simulink model "IEEE34bus_v2019b_Phasor_DPL_ZIPload"  (R2019b)
settings: Solver=VariableStepAuto  StartTime=0.0  StopTime=100  FixedStep=Ts  RelTol=1e-3
InitFcn:
  | a=1; % Loading Factor
  | Ts=0.1;% For Delay Blocks in Voltage Regulator Controls
  | 
  | % Simulation data for the IEEE 34 Node Test Feeder model
  | mi2km = 1.60934;%  miles to km conversion
  | ft2km = 0.0003048; % feet to km conversion
  | ms2F = 1*1e-6/(2*pi*60);% microsiemens to Farads conversion
  | 
  | %% Configuration 300 - series reactance - ohm/mile
  | R_300 = [1.3368 0.2101 0.2130;0.2101 1.3238 0.2066;0.2130 0.2066 1.3294];
  | X_300 = [1.3343 0.5779 0.5015;0.5779 1.3569 0.4591;0.5015 0.4591 1.3471];
  | % charging susceptance - microsiemens/mile
  | B_300 = [5.3350 -1.5313 -0.9943;-1.5313 5.0979 -0.6212;-0.9943 -0.6212 4.8880];
  | 
  | R_300 = R_300/mi2km;
  | L_300 = (X_300/(2*pi*60))/mi2km;
  | C_300 =(B_300*ms2F)/mi2km;
  | 
  | %% Configuration 301 - series reactance - ohm/mile
  | R_301 = [1.9300 0.2327 0.2359;0.2327 1.9157 0.2288;0.2359 0.2288 1.9219];
  | X_301 = [1.4115 0.6442 0.5691;0.6442 1.4281 0.5238;0.5691 0.5238 1.4209];
  | % charging susceptance - microsiemens/mile
  | B_301 = [5.1207 -1.4364 -0.9402;-1.4364 4.9055 -0.5951;-0.9402 -0.5951 4.7154];
  | 
  | R_301 = R_301/mi2km;
  | L_301 = (X_301/(2*pi*60))/mi2km;
  | C_301 =(B_301*ms2F)/mi2km;
  | 
  | 
  | %% Configuration 302 - series reactance - ohm/mile
  | R_302 = [2.7995 0 0;0 0 0;0 0 0];
  | X_302 = [1.4855 0 0;0 0 0;0 0 0];
  | % charging susceptance - microsiemens/mile
  | B_302 = [4.2251 0 0;0 0 0;0 0 0];
  | 
  | R_302 = R_302/mi2km;
  | L_302 = (X_302/(2*pi*60))/mi2km;
  | C_302 =(B_302*ms2F)/mi2km;
  | 
  | %% Configuration 303 - series reactance - ohm/mile
  | R_303 = [0 0 0;0 2.7995 0;0 0 0];
  | X_303 = [0 0 0;0 1.4855 0;0 0 0];
  | % charging susceptance - microsiemens/mile
  | B_303 = [0 0 0;0 4.2251 0;0 0 0];
  | 
  | R_303 = R_303/mi2km;
  | L_303 = (X_303/(2*pi*60))/mi2km;
  | C_303 =(B_303*ms2F)/mi2km;
  | 
  | %% Configuration 303 - series reactance - ohm/mile
  | R_304 = [0 0 0;0 1.9217 0;0 0 0];
  | X_304 = [0 0 0;0 1.4212 0;0 0 0];
  | % charging susceptance - microsiemens/mile
  | B_304 = [0 0 0;0 4.3637 0;0 0 0];
  | 
  | R_304 = R_304/mi2km;
  | L_304 = (X_304/(2*pi*60))/mi2km;
  | C_304 =(B_304*ms2F)/mi2km;
undefined symbols (not defined in the file): find_system, j
libraries: powerlib x471, powerlib_meascontrol x22
(part 7 of 9)

== system IEEE34bus_v2019b_Phasor_DPL_ZIPload/Regulator 1/Single Phase SVR_B/Voltage Regulator Control/Voltage regulator ==
  Vmes (pu) : Inport
  Ready : Inport  Port=2
  RegOn : Inport  Port=3
  Dead Zone : DeadZone  LowerValue=-DeadBand/2  UpperValue=+DeadBand/2  SaturateOnIntegerOverflow=on
  Discrete Variable Time Delay : powerlib_meascontrol/Additional Components/Discrete Variable Time Delay  MaxDelay=3/60+Ts  InitialValue=1  Ts=Ts  DFT=on
      settings: SourceProductName=Simscape Electrical  SourceProductBaseCode=PS
  Logical Operator : Logic  AllPortsSameDT=off
  Logical Operator1 : Logic  AllPortsSameDT=off
  On Delay : powerlib_meascontrol/Logic/On Delay  DelayType=On delay  delay=TimeDelay  ic=0  Ts=Ts
      settings: SourceProductName=Simscape Electrical
  On Delay1 : powerlib_meascontrol/Logic/On Delay  DelayType=On delay  delay=TimeDelay  ic=0  Ts=Ts
      settings: SourceProductName=Simscape Electrical
  Relational Operator : RelationalOperator  Operator=>  RndMeth=Nearest
  Relational Operator1 : RelationalOperator  Operator=<  RndMeth=Nearest
  Sum : Sum  Inputs=|+-  SaturateOnIntegerOverflow=on
  Switch : Switch  Threshold=1.5  SaturateOnIntegerOverflow=on
  Vref : Constant  Value=Vref
  Vref1 : Constant  Value=0
  Vref2 : Constant  Value=0
  Vref3 : Constant  Value=0
  Vref4 : Constant  Value=3/60
  Up : Outport  VectorParamsAs1DForOutWhenUnconnected=off
  Down : Outport  Port=2  VectorParamsAs1DForOutWhenUnconnected=off
  wires:
  Vref2/1 -> Switch/3
  RegOn/1 -> Switch/2
  Switch/1 -> Dead Zone/1
  Sum/1 -> Switch/1
  Vref/1 -> Sum/1
  Vmes (pu)/1 -> Sum/2
  Dead Zone/1 -> Relational Operator1/1, Relational Operator/1
  Vref1/1 -> Relational Operator/2
  Relational Operator/1 -> Logical Operator/1
  Ready/1 -> Discrete Variable Time Delay/1
  Logical Operator/1 -> On Delay/1
  On Delay/1 -> Up/1
  Relational Operator1/1 -> Logical Operator1/2
  Logical Operator1/1 -> On Delay1/1
  On Delay1/1 -> Down/1
  Vref3/1 -> Relational Operator1/2
  Discrete Variable Time Delay/1 -> Logical Operator1/1, Logical Operator/2
  Vref4/1 -> Discrete Variable Time Delay/2

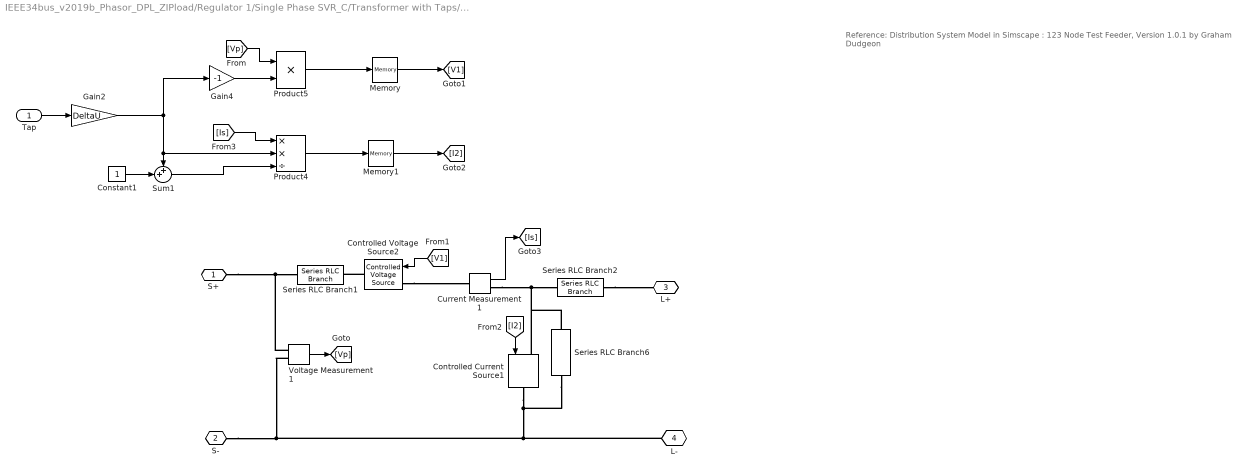
== system IEEE34bus_v2019b_Phasor_DPL_ZIPload/Regulator 1/Single Phase SVR_C/Transformer with Taps/Tap Changing Transformer ==
  note: Reference:
      | Distribution System Model in Simscape : 123 Node Test Feeder, Version 1.0.1  by Graham Dudgeon
  Tap : Inport
  Constant1 : Constant
  Controlled Current Source1 : powerlib/Electrical Sources/Controlled Current Source  Initialize=off  Source_Type=AC  Amplitude=0  Phase=0  Frequency=0  Measurements=None
      settings: SourceProductName=Simscape Electrical
  Controlled Voltage Source2 : powerlib/Electrical Sources/Controlled Voltage Source  Initialize=off  Source_Type=AC  Amplitude=0  Phase=0  Frequency=0  Measurements=None
      settings: SourceProductName=Simscape Electrical
  Current Measurement1 : powerlib/Measurements/Current Measurement  PhasorSimulation=on  OutputType=Complex  PSBequivalent=0
      settings: SourceProductName=Simscape Electrical
  Gain2 : Gain  Gain=DeltaU
  Gain4 : Gain  Gain=-1
  Memory : Memory
  Memory1 : Memory
  Product4 : Product  Inputs=**/  RndMeth=Zero
  Product5 : Product  Inputs=**  RndMeth=Zero
  Series RLC Branch1 : powerlib/Elements/Series RLC Branch  LConnTagsString=__new0  RConnTagsString=__new0  BranchType=R  Resistance=1e-6  Inductance=1e-3  SetiL0=off  InitialCurrent=0  Capacitance=1e-6  Setx0=off  InitialVoltage=0  Measurements=None
      settings: SourceProductName=Simscape Electrical
  Series RLC Branch2 : powerlib/Elements/Series RLC Branch  LConnTagsString=__new0  RConnTagsString=__new0  BranchType=R  Resistance=1e-6  Inductance=1e-3  SetiL0=off  InitialCurrent=0  Capacitance=1e-6  Setx0=off  InitialVoltage=0  Measurements=None
      settings: SourceProductName=Simscape Electrical
  Series RLC Branch6 : powerlib/Elements/Series RLC Branch  LConnTagsString=__new0  RConnTagsString=__new0  BranchType=R  Resistance=1e6  Inductance=1e-3  SetiL0=off  InitialCurrent=0  Capacitance=1e-6  Setx0=off  InitialVoltage=0  Measurements=None
      settings: SourceProductName=Simscape Electrical
  Sum1 : Sum  Inputs=++|
  Voltage Measurement1 : powerlib/Measurements/Voltage Measurement  PhasorSimulation=on  OutputType=Complex  PSBequivalent=0
      settings: SourceProductName=Simscape Electrical
  S+ : PMIOPort  Side=Left
  S- : PMIOPort  Port=2  Side=Left
  L+ : PMIOPort  Port=3  Side=Right
  L- : PMIOPort  Port=4  Side=Right
  wires:
  Sum1/1 -> Product4/3
  [I2] -> Controlled Current Source1/1
  [V1] -> Controlled Voltage Source2/1
  Constant1/1 -> Sum1/2
  Product5/1 -> Memory/1
  Product4/1 -> Memory1/1
  [Is] -> Product4/1
  Current Measurement1/1 -> [Is]
  Tap/1 -> Gain2/1
  Gain2/1 -> Sum1/1, Product4/2, Gain4/1
  Gain4/1 -> Product5/2
  [Vp] -> Product5/1
  Voltage Measurement1/1 -> [Vp]
  Memory/1 -> [V1]
  Memory1/1 -> [I2]
  connections:
  Series RLC Branch6/LConn1 -- Controlled Current Source1/RConn1 -- S-/RConn1 -- Voltage Measurement1/LConn2 -- L-/RConn1
  Controlled Voltage Source2/RConn1 -- Series RLC Branch1/LConn1
  Current Measurement1/RConn1 -- Series RLC Branch6/RConn1 -- Controlled Current Source1/LConn1 -- Series RLC Branch2/RConn1
  Controlled Voltage Source2/LConn1 -- Current Measurement1/LConn1
  Voltage Measurement1/LConn1 -- Series RLC Branch1/RConn1 -- S+/RConn1
  Series RLC Branch2/LConn1 -- L+/RConn1

== system IEEE34bus_v2019b_Phasor_DPL_ZIPload/Regulator 1/Single Phase SVR_C/Voltage Regulator Control/Tap Changer Control ==
  "Up " : Inport
  "Down " : Inport  Port=2
  Constant : Constant  Value=-1
  Constant1 : Constant
  Determine tap position : Subsystem
  Edge Detector : Subsystem  DialogController=POWERSYS.PowerSysDialog  mask(Edge Detector){model=Rising, ic=0}
      mask prompts: model "Edge:"; ic "Input at t = -eps:"
      mask help:
      | This block compares its present input to its previous input.
      |
      | If the input  is a logic signal (TRUE (1) or FALSE (0), the output is a one-step boolean signal TRUE  when  the specified edge (Rising, Falling or Either)  is detected.
      |
      | This block can also be used to detect the slope polarity of a continuous signal. For example, if the specified edge is  "Rising", the output is TRUE as long as the slope of the input signal is positive.
      |
      | The input value at time preceding t=0 is specified by the parameter "Input at t=-eps"
      mask init: same as IEEE34bus_v2019b_Phasor_DPL_ZIPload/Regulator 1/Single Phase SVR_A/Voltage Regulator Control/Tap Changer Control/Edge Detector
      mask Help: This block is part of a subset of blocks in the Extras library that does not have documentation associated with it, other than the block mask description.
      mask TypeOptions model: Rising | Falling | Either
      mask Display: plot(0,0,100,100, X1,Y1,X2,Y2,X3,Y3,X4,Y4);
  Logical Operator : Logic  Operator=OR  AllPortsSameDT=off
  Logical Operator1 : Logic  AllPortsSameDT=off
  Mechanical Delay : TransportDelay  DelayTime=MecDelay  InitialOutput=InitialPosition  BufferSize=5120
  Memory : Memory  InitialCondition=1  InheritSampleTime=on
  Relational Operator : RelationalOperator  Operator===  OutDataTypeStr=float('double')  RndMeth=Nearest
  Switch : Switch  Threshold=0.5  SaturateOnIntegerOverflow=on
  TapNo : Outport  VectorParamsAs1DForOutWhenUnconnected=off
  Ready : Outport  Port=2  VectorParamsAs1DForOutWhenUnconnected=off
  wires:
  Mechanical Delay/1 -> TapNo/1, Relational Operator/2
  Logical Operator1/1 -> Determine tap position/Trigger
  "Up "/1 -> Logical Operator/1
  "Down "/1 -> Logical Operator/2, Switch/2
  Constant/1 -> Switch/1
  Constant1/1 -> Switch/3
  Switch/1 -> Determine tap position/1(NewTap)
  Determine tap position/1(TapNo) -> Mechanical Delay/1, Relational Operator/1
  Relational Operator/1 -> Memory/1
  Memory/1 -> Logical Operator1/1, Ready/1
  Logical Operator/1 -> Edge Detector/1(In)
  Edge Detector/1(Out) -> Logical Operator1/2

== system IEEE34bus_v2019b_Phasor_DPL_ZIPload/Regulator 1/Single Phase SVR_C/Voltage Regulator Control/Voltage regulator ==
  Vmes (pu) : Inport
  Ready : Inport  Port=2
  RegOn : Inport  Port=3
  Dead Zone : DeadZone  LowerValue=-DeadBand/2  UpperValue=+DeadBand/2  SaturateOnIntegerOverflow=on
  Discrete Variable Time Delay : powerlib_meascontrol/Additional Components/Discrete Variable Time Delay  MaxDelay=3/60+Ts  InitialValue=1  Ts=Ts  DFT=on
      settings: SourceProductName=Simscape Electrical  SourceProductBaseCode=PS
  Logical Operator : Logic  AllPortsSameDT=off
  Logical Operator1 : Logic  AllPortsSameDT=off
  On Delay : powerlib_meascontrol/Logic/On Delay  DelayType=On delay  delay=TimeDelay  ic=0  Ts=Ts
      settings: SourceProductName=Simscape Electrical
  On Delay1 : powerlib_meascontrol/Logic/On Delay  DelayType=On delay  delay=TimeDelay  ic=0  Ts=Ts
      settings: SourceProductName=Simscape Electrical
  Relational Operator : RelationalOperator  Operator=>  RndMeth=Nearest
  Relational Operator1 : RelationalOperator  Operator=<  RndMeth=Nearest
  Sum : Sum  Inputs=|+-  SaturateOnIntegerOverflow=on
  Switch : Switch  Threshold=1.5  SaturateOnIntegerOverflow=on
  Vref : Constant  Value=Vref
  Vref1 : Constant  Value=0
  Vref2 : Constant  Value=0
  Vref3 : Constant  Value=0
  Vref4 : Constant  Value=3/60
  Up : Outport  VectorParamsAs1DForOutWhenUnconnected=off
  Down : Outport  Port=2  VectorParamsAs1DForOutWhenUnconnected=off
  wires:
  Vref2/1 -> Switch/3
  RegOn/1 -> Switch/2
  Switch/1 -> Dead Zone/1
  Sum/1 -> Switch/1
  Vref/1 -> Sum/1
  Vmes (pu)/1 -> Sum/2
  Dead Zone/1 -> Relational Operator1/1, Relational Operator/1
  Vref1/1 -> Relational Operator/2
  Relational Operator/1 -> Logical Operator/1
  Ready/1 -> Discrete Variable Time Delay/1
  Logical Operator/1 -> On Delay/1
  On Delay/1 -> Up/1
  Relational Operator1/1 -> Logical Operator1/2
  Logical Operator1/1 -> On Delay1/1
  On Delay1/1 -> Down/1
  Vref3/1 -> Relational Operator1/2
  Discrete Variable Time Delay/1 -> Logical Operator1/1, Logical Operator/2
  Vref4/1 -> Discrete Variable Time Delay/2

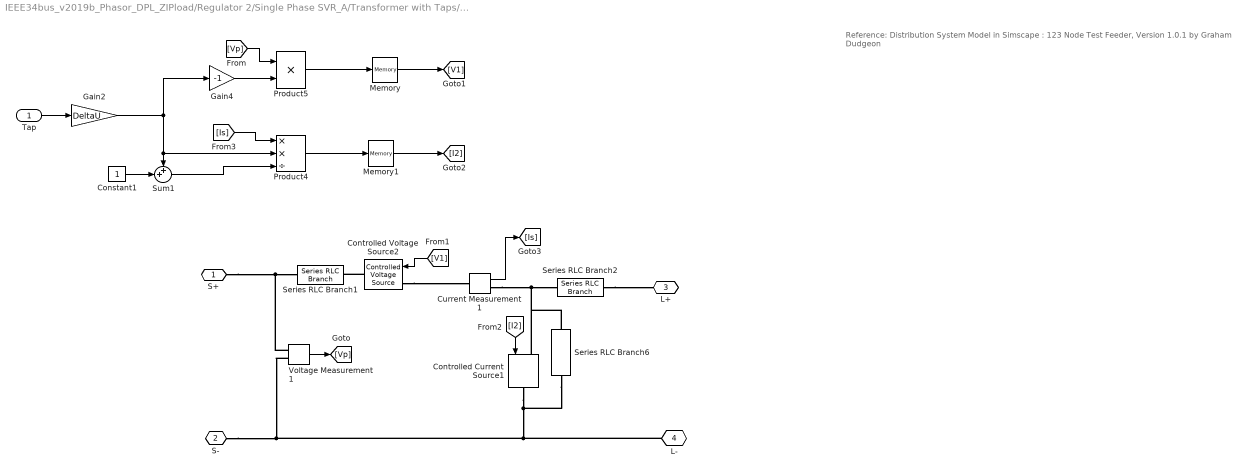
== system IEEE34bus_v2019b_Phasor_DPL_ZIPload/Regulator 2/Single Phase SVR_A/Transformer with Taps/Tap Changing Transformer ==
  note: Reference:
      | Distribution System Model in Simscape : 123 Node Test Feeder, Version 1.0.1  by Graham Dudgeon
  Tap : Inport
  Constant1 : Constant
  Controlled Current Source1 : powerlib/Electrical Sources/Controlled Current Source  Initialize=off  Source_Type=AC  Amplitude=0  Phase=0  Frequency=0  Measurements=None
      settings: SourceProductName=Simscape Electrical
  Controlled Voltage Source2 : powerlib/Electrical Sources/Controlled Voltage Source  Initialize=off  Source_Type=AC  Amplitude=0  Phase=0  Frequency=0  Measurements=None
      settings: SourceProductName=Simscape Electrical
  Current Measurement1 : powerlib/Measurements/Current Measurement  PhasorSimulation=on  OutputType=Complex  PSBequivalent=0
      settings: SourceProductName=Simscape Electrical
  Gain2 : Gain  Gain=DeltaU
  Gain4 : Gain  Gain=-1
  Memory : Memory
  Memory1 : Memory
  Product4 : Product  Inputs=**/  RndMeth=Zero
  Product5 : Product  Inputs=**  RndMeth=Zero
  Series RLC Branch1 : powerlib/Elements/Series RLC Branch  LConnTagsString=__new0  RConnTagsString=__new0  BranchType=R  Resistance=1e-6  Inductance=1e-3  SetiL0=off  InitialCurrent=0  Capacitance=1e-6  Setx0=off  InitialVoltage=0  Measurements=None
      settings: SourceProductName=Simscape Electrical
  Series RLC Branch2 : powerlib/Elements/Series RLC Branch  LConnTagsString=__new0  RConnTagsString=__new0  BranchType=R  Resistance=1e-6  Inductance=1e-3  SetiL0=off  InitialCurrent=0  Capacitance=1e-6  Setx0=off  InitialVoltage=0  Measurements=None
      settings: SourceProductName=Simscape Electrical
  Series RLC Branch6 : powerlib/Elements/Series RLC Branch  LConnTagsString=__new0  RConnTagsString=__new0  BranchType=R  Resistance=1e6  Inductance=1e-3  SetiL0=off  InitialCurrent=0  Capacitance=1e-6  Setx0=off  InitialVoltage=0  Measurements=None
      settings: SourceProductName=Simscape Electrical
  Sum1 : Sum  Inputs=++|
  Voltage Measurement1 : powerlib/Measurements/Voltage Measurement  PhasorSimulation=on  OutputType=Complex  PSBequivalent=0
      settings: SourceProductName=Simscape Electrical
  S+ : PMIOPort  Side=Left
  S- : PMIOPort  Port=2  Side=Left
  L+ : PMIOPort  Port=3  Side=Right
  L- : PMIOPort  Port=4  Side=Right
  wires:
  Sum1/1 -> Product4/3
  [I2] -> Controlled Current Source1/1
  [V1] -> Controlled Voltage Source2/1
  Constant1/1 -> Sum1/2
  Product5/1 -> Memory/1
  Product4/1 -> Memory1/1
  [Is] -> Product4/1
  Current Measurement1/1 -> [Is]
  Tap/1 -> Gain2/1
  Gain2/1 -> Sum1/1, Product4/2, Gain4/1
  Gain4/1 -> Product5/2
  [Vp] -> Product5/1
  Voltage Measurement1/1 -> [Vp]
  Memory/1 -> [V1]
  Memory1/1 -> [I2]
  connections:
  Series RLC Branch6/LConn1 -- Controlled Current Source1/RConn1 -- S-/RConn1 -- Voltage Measurement1/LConn2 -- L-/RConn1
  Controlled Voltage Source2/RConn1 -- Series RLC Branch1/LConn1
  Current Measurement1/RConn1 -- Series RLC Branch6/RConn1 -- Controlled Current Source1/LConn1 -- Series RLC Branch2/RConn1
  Controlled Voltage Source2/LConn1 -- Current Measurement1/LConn1
  Voltage Measurement1/LConn1 -- Series RLC Branch1/RConn1 -- S+/RConn1
  Series RLC Branch2/LConn1 -- L+/RConn1

== system IEEE34bus_v2019b_Phasor_DPL_ZIPload/Regulator 2/Single Phase SVR_A/Voltage Regulator Control/Tap Changer Control ==
  "Up " : Inport
  "Down " : Inport  Port=2
  Constant : Constant  Value=-1
  Constant1 : Constant
  Determine tap position : Subsystem
  Edge Detector : Subsystem  DialogController=POWERSYS.PowerSysDialog  mask(Edge Detector){model=Rising, ic=0}
      mask prompts: model "Edge:"; ic "Input at t = -eps:"
      mask help:
      | This block compares its present input to its previous input.
      |
      | If the input  is a logic signal (TRUE (1) or FALSE (0), the output is a one-step boolean signal TRUE  when  the specified edge (Rising, Falling or Either)  is detected.
      |
      | This block can also be used to detect the slope polarity of a continuous signal. For example, if the specified edge is  "Rising", the output is TRUE as long as the slope of the input signal is positive.
      |
      | The input value at time preceding t=0 is specified by the parameter "Input at t=-eps"
      mask init: same as IEEE34bus_v2019b_Phasor_DPL_ZIPload/Regulator 1/Single Phase SVR_A/Voltage Regulator Control/Tap Changer Control/Edge Detector
      mask Help: This block is part of a subset of blocks in the Extras library that does not have documentation associated with it, other than the block mask description.
      mask TypeOptions model: Rising | Falling | Either
      mask Display: plot(0,0,100,100, X1,Y1,X2,Y2,X3,Y3,X4,Y4);
  Logical Operator : Logic  Operator=OR  AllPortsSameDT=off
  Logical Operator1 : Logic  AllPortsSameDT=off
  Mechanical Delay : TransportDelay  DelayTime=MecDelay  InitialOutput=InitialPosition  BufferSize=5120
  Memory : Memory  InitialCondition=1  InheritSampleTime=on
  Relational Operator : RelationalOperator  Operator===  OutDataTypeStr=float('double')  RndMeth=Nearest
  Switch : Switch  Threshold=0.5  SaturateOnIntegerOverflow=on
  TapNo : Outport  VectorParamsAs1DForOutWhenUnconnected=off
  Ready : Outport  Port=2  VectorParamsAs1DForOutWhenUnconnected=off
  wires:
  Mechanical Delay/1 -> TapNo/1, Relational Operator/2
  Logical Operator1/1 -> Determine tap position/Trigger
  "Up "/1 -> Logical Operator/1
  "Down "/1 -> Logical Operator/2, Switch/2
  Constant/1 -> Switch/1
  Constant1/1 -> Switch/3
  Switch/1 -> Determine tap position/1(NewTap)
  Determine tap position/1(TapNo) -> Mechanical Delay/1, Relational Operator/1
  Relational Operator/1 -> Memory/1
  Memory/1 -> Logical Operator1/1, Ready/1
  Logical Operator/1 -> Edge Detector/1(In)
  Edge Detector/1(Out) -> Logical Operator1/2

== system IEEE34bus_v2019b_Phasor_DPL_ZIPload/Regulator 2/Single Phase SVR_A/Voltage Regulator Control/Voltage regulator ==
  Vmes (pu) : Inport
  Ready : Inport  Port=2
  RegOn : Inport  Port=3
  Dead Zone : DeadZone  LowerValue=-DeadBand/2  UpperValue=+DeadBand/2  SaturateOnIntegerOverflow=on
  Discrete Variable Time Delay : powerlib_meascontrol/Additional Components/Discrete Variable Time Delay  MaxDelay=3/60+Ts  InitialValue=1  Ts=Ts  DFT=on
      settings: SourceProductName=Simscape Electrical  SourceProductBaseCode=PS
  Logical Operator : Logic  AllPortsSameDT=off
  Logical Operator1 : Logic  AllPortsSameDT=off
  On Delay : powerlib_meascontrol/Logic/On Delay  DelayType=On delay  delay=TimeDelay  ic=0  Ts=Ts
      settings: SourceProductName=Simscape Electrical
  On Delay1 : powerlib_meascontrol/Logic/On Delay  DelayType=On delay  delay=TimeDelay  ic=0  Ts=Ts
      settings: SourceProductName=Simscape Electrical
  Relational Operator : RelationalOperator  Operator=>  RndMeth=Nearest
  Relational Operator1 : RelationalOperator  Operator=<  RndMeth=Nearest
  Sum : Sum  Inputs=|+-  SaturateOnIntegerOverflow=on
  Switch : Switch  Threshold=1.5  SaturateOnIntegerOverflow=on
  Vref : Constant  Value=Vref
  Vref1 : Constant  Value=0
  Vref2 : Constant  Value=0
  Vref3 : Constant  Value=0
  Vref4 : Constant  Value=3/60
  Up : Outport  VectorParamsAs1DForOutWhenUnconnected=off
  Down : Outport  Port=2  VectorParamsAs1DForOutWhenUnconnected=off
  wires:
  Vref2/1 -> Switch/3
  RegOn/1 -> Switch/2
  Switch/1 -> Dead Zone/1
  Sum/1 -> Switch/1
  Vref/1 -> Sum/1
  Vmes (pu)/1 -> Sum/2
  Dead Zone/1 -> Relational Operator1/1, Relational Operator/1
  Vref1/1 -> Relational Operator/2
  Relational Operator/1 -> Logical Operator/1
  Ready/1 -> Discrete Variable Time Delay/1
  Logical Operator/1 -> On Delay/1
  On Delay/1 -> Up/1
  Relational Operator1/1 -> Logical Operator1/2
  Logical Operator1/1 -> On Delay1/1
  On Delay1/1 -> Down/1
  Vref3/1 -> Relational Operator1/2
  Discrete Variable Time Delay/1 -> Logical Operator1/1, Logical Operator/2
  Vref4/1 -> Discrete Variable Time Delay/2

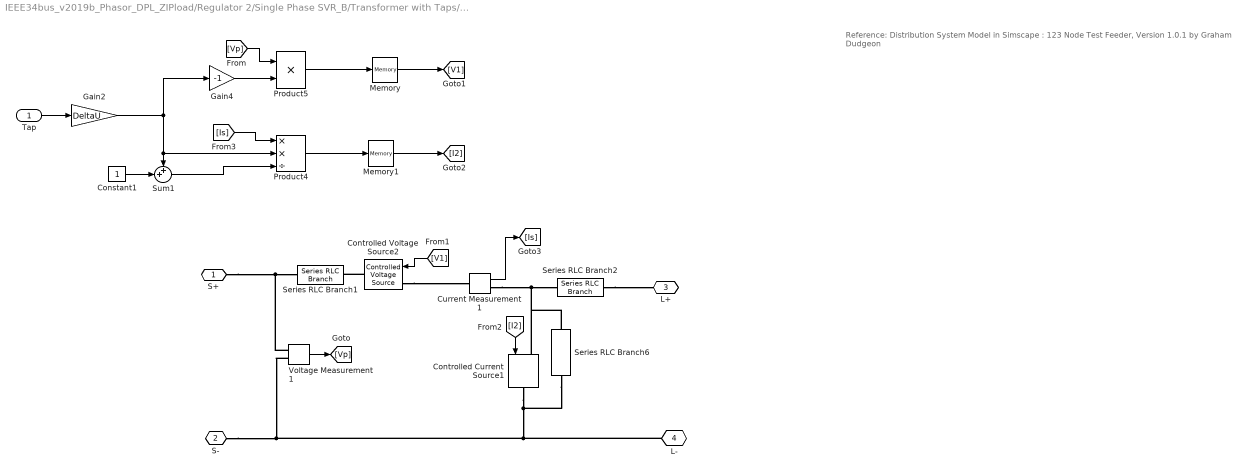
== system IEEE34bus_v2019b_Phasor_DPL_ZIPload/Regulator 2/Single Phase SVR_B/Transformer with Taps/Tap Changing Transformer ==
  note: Reference:
      | Distribution System Model in Simscape : 123 Node Test Feeder, Version 1.0.1  by Graham Dudgeon
  Tap : Inport
  Constant1 : Constant
  Controlled Current Source1 : powerlib/Electrical Sources/Controlled Current Source  Initialize=off  Source_Type=AC  Amplitude=0  Phase=0  Frequency=0  Measurements=None
      settings: SourceProductName=Simscape Electrical
  Controlled Voltage Source2 : powerlib/Electrical Sources/Controlled Voltage Source  Initialize=off  Source_Type=AC  Amplitude=0  Phase=0  Frequency=0  Measurements=None
      settings: SourceProductName=Simscape Electrical
  Current Measurement1 : powerlib/Measurements/Current Measurement  PhasorSimulation=on  OutputType=Complex  PSBequivalent=0
      settings: SourceProductName=Simscape Electrical
  Gain2 : Gain  Gain=DeltaU
  Gain4 : Gain  Gain=-1
  Memory : Memory
  Memory1 : Memory
  Product4 : Product  Inputs=**/  RndMeth=Zero
  Product5 : Product  Inputs=**  RndMeth=Zero
  Series RLC Branch1 : powerlib/Elements/Series RLC Branch  LConnTagsString=__new0  RConnTagsString=__new0  BranchType=R  Resistance=1e-6  Inductance=1e-3  SetiL0=off  InitialCurrent=0  Capacitance=1e-6  Setx0=off  InitialVoltage=0  Measurements=None
      settings: SourceProductName=Simscape Electrical
  Series RLC Branch2 : powerlib/Elements/Series RLC Branch  LConnTagsString=__new0  RConnTagsString=__new0  BranchType=R  Resistance=1e-6  Inductance=1e-3  SetiL0=off  InitialCurrent=0  Capacitance=1e-6  Setx0=off  InitialVoltage=0  Measurements=None
      settings: SourceProductName=Simscape Electrical
  Series RLC Branch6 : powerlib/Elements/Series RLC Branch  LConnTagsString=__new0  RConnTagsString=__new0  BranchType=R  Resistance=1e6  Inductance=1e-3  SetiL0=off  InitialCurrent=0  Capacitance=1e-6  Setx0=off  InitialVoltage=0  Measurements=None
      settings: SourceProductName=Simscape Electrical
  Sum1 : Sum  Inputs=++|
  Voltage Measurement1 : powerlib/Measurements/Voltage Measurement  PhasorSimulation=on  OutputType=Complex  PSBequivalent=0
      settings: SourceProductName=Simscape Electrical
  S+ : PMIOPort  Side=Left
  S- : PMIOPort  Port=2  Side=Left
  L+ : PMIOPort  Port=3  Side=Right
  L- : PMIOPort  Port=4  Side=Right
  wires:
  Sum1/1 -> Product4/3
  [I2] -> Controlled Current Source1/1
  [V1] -> Controlled Voltage Source2/1
  Constant1/1 -> Sum1/2
  Product5/1 -> Memory/1
  Product4/1 -> Memory1/1
  [Is] -> Product4/1
  Current Measurement1/1 -> [Is]
  Tap/1 -> Gain2/1
  Gain2/1 -> Sum1/1, Product4/2, Gain4/1
  Gain4/1 -> Product5/2
  [Vp] -> Product5/1
  Voltage Measurement1/1 -> [Vp]
  Memory/1 -> [V1]
  Memory1/1 -> [I2]
  connections:
  Series RLC Branch6/LConn1 -- Controlled Current Source1/RConn1 -- S-/RConn1 -- Voltage Measurement1/LConn2 -- L-/RConn1
  Controlled Voltage Source2/RConn1 -- Series RLC Branch1/LConn1
  Current Measurement1/RConn1 -- Series RLC Branch6/RConn1 -- Controlled Current Source1/LConn1 -- Series RLC Branch2/RConn1
  Controlled Voltage Source2/LConn1 -- Current Measurement1/LConn1
  Voltage Measurement1/LConn1 -- Series RLC Branch1/RConn1 -- S+/RConn1
  Series RLC Branch2/LConn1 -- L+/RConn1

== system IEEE34bus_v2019b_Phasor_DPL_ZIPload/Regulator 2/Single Phase SVR_B/Voltage Regulator Control/Tap Changer Control ==
  "Up " : Inport
  "Down " : Inport  Port=2
  Constant : Constant  Value=-1
  Constant1 : Constant
  Determine tap position : Subsystem
  Edge Detector : Subsystem  DialogController=POWERSYS.PowerSysDialog  mask(Edge Detector){model=Rising, ic=0}
      mask prompts: model "Edge:"; ic "Input at t = -eps:"
      mask help:
      | This block compares its present input to its previous input.
      |
      | If the input  is a logic signal (TRUE (1) or FALSE (0), the output is a one-step boolean signal TRUE  when  the specified edge (Rising, Falling or Either)  is detected.
      |
      | This block can also be used to detect the slope polarity of a continuous signal. For example, if the specified edge is  "Rising", the output is TRUE as long as the slope of the input signal is positive.
      |
      | The input value at time preceding t=0 is specified by the parameter "Input at t=-eps"
      mask init: same as IEEE34bus_v2019b_Phasor_DPL_ZIPload/Regulator 1/Single Phase SVR_A/Voltage Regulator Control/Tap Changer Control/Edge Detector
      mask Help: This block is part of a subset of blocks in the Extras library that does not have documentation associated with it, other than the block mask description.
      mask TypeOptions model: Rising | Falling | Either
      mask Display: plot(0,0,100,100, X1,Y1,X2,Y2,X3,Y3,X4,Y4);
  Logical Operator : Logic  Operator=OR  AllPortsSameDT=off
  Logical Operator1 : Logic  AllPortsSameDT=off
  Mechanical Delay : TransportDelay  DelayTime=MecDelay  InitialOutput=InitialPosition  BufferSize=5120
  Memory : Memory  InitialCondition=1  InheritSampleTime=on
  Relational Operator : RelationalOperator  Operator===  OutDataTypeStr=float('double')  RndMeth=Nearest
  Switch : Switch  Threshold=0.5  SaturateOnIntegerOverflow=on
  TapNo : Outport  VectorParamsAs1DForOutWhenUnconnected=off
  Ready : Outport  Port=2  VectorParamsAs1DForOutWhenUnconnected=off
  wires:
  Mechanical Delay/1 -> TapNo/1, Relational Operator/2
  Logical Operator1/1 -> Determine tap position/Trigger
  "Up "/1 -> Logical Operator/1
  "Down "/1 -> Logical Operator/2, Switch/2
  Constant/1 -> Switch/1
  Constant1/1 -> Switch/3
  Switch/1 -> Determine tap position/1(NewTap)
  Determine tap position/1(TapNo) -> Mechanical Delay/1, Relational Operator/1
  Relational Operator/1 -> Memory/1
  Memory/1 -> Logical Operator1/1, Ready/1
  Logical Operator/1 -> Edge Detector/1(In)
  Edge Detector/1(Out) -> Logical Operator1/2

== system IEEE34bus_v2019b_Phasor_DPL_ZIPload/Regulator 2/Single Phase SVR_B/Voltage Regulator Control/Voltage regulator ==
  Vmes (pu) : Inport
  Ready : Inport  Port=2
  RegOn : Inport  Port=3
  Dead Zone : DeadZone  LowerValue=-DeadBand/2  UpperValue=+DeadBand/2  SaturateOnIntegerOverflow=on
  Discrete Variable Time Delay : powerlib_meascontrol/Additional Components/Discrete Variable Time Delay  MaxDelay=3/60+Ts  InitialValue=1  Ts=Ts  DFT=on
      settings: SourceProductName=Simscape Electrical  SourceProductBaseCode=PS
  Logical Operator : Logic  AllPortsSameDT=off
  Logical Operator1 : Logic  AllPortsSameDT=off
  On Delay : powerlib_meascontrol/Logic/On Delay  DelayType=On delay  delay=TimeDelay  ic=0  Ts=Ts
      settings: SourceProductName=Simscape Electrical
  On Delay1 : powerlib_meascontrol/Logic/On Delay  DelayType=On delay  delay=TimeDelay  ic=0  Ts=Ts
      settings: SourceProductName=Simscape Electrical
  Relational Operator : RelationalOperator  Operator=>  RndMeth=Nearest
  Relational Operator1 : RelationalOperator  Operator=<  RndMeth=Nearest
  Sum : Sum  Inputs=|+-  SaturateOnIntegerOverflow=on
  Switch : Switch  Threshold=1.5  SaturateOnIntegerOverflow=on
  Vref : Constant  Value=Vref
  Vref1 : Constant  Value=0
  Vref2 : Constant  Value=0
  Vref3 : Constant  Value=0
  Vref4 : Constant  Value=3/60
  Up : Outport  VectorParamsAs1DForOutWhenUnconnected=off
  Down : Outport  Port=2  VectorParamsAs1DForOutWhenUnconnected=off
  wires:
  Vref2/1 -> Switch/3
  RegOn/1 -> Switch/2
  Switch/1 -> Dead Zone/1
  Sum/1 -> Switch/1
  Vref/1 -> Sum/1
  Vmes (pu)/1 -> Sum/2
  Dead Zone/1 -> Relational Operator1/1, Relational Operator/1
  Vref1/1 -> Relational Operator/2
  Relational Operator/1 -> Logical Operator/1
  Ready/1 -> Discrete Variable Time Delay/1
  Logical Operator/1 -> On Delay/1
  On Delay/1 -> Up/1
  Relational Operator1/1 -> Logical Operator1/2
  Logical Operator1/1 -> On Delay1/1
  On Delay1/1 -> Down/1
  Vref3/1 -> Relational Operator1/2
  Discrete Variable Time Delay/1 -> Logical Operator1/1, Logical Operator/2
  Vref4/1 -> Discrete Variable Time Delay/2

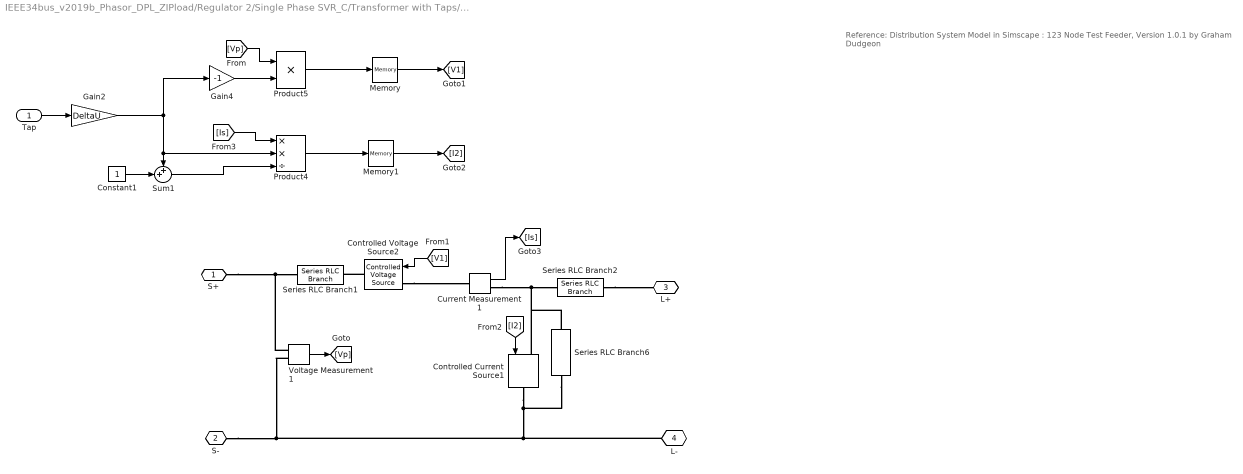
== system IEEE34bus_v2019b_Phasor_DPL_ZIPload/Regulator 2/Single Phase SVR_C/Transformer with Taps/Tap Changing Transformer ==
  note: Reference:
      | Distribution System Model in Simscape : 123 Node Test Feeder, Version 1.0.1  by Graham Dudgeon
  Tap : Inport
  Constant1 : Constant
  Controlled Current Source1 : powerlib/Electrical Sources/Controlled Current Source  Initialize=off  Source_Type=AC  Amplitude=0  Phase=0  Frequency=0  Measurements=None
      settings: SourceProductName=Simscape Electrical
  Controlled Voltage Source2 : powerlib/Electrical Sources/Controlled Voltage Source  Initialize=off  Source_Type=AC  Amplitude=0  Phase=0  Frequency=0  Measurements=None
      settings: SourceProductName=Simscape Electrical
  Current Measurement1 : powerlib/Measurements/Current Measurement  PhasorSimulation=on  OutputType=Complex  PSBequivalent=0
      settings: SourceProductName=Simscape Electrical
  Gain2 : Gain  Gain=DeltaU
  Gain4 : Gain  Gain=-1
  Memory : Memory
  Memory1 : Memory
  Product4 : Product  Inputs=**/  RndMeth=Zero
  Product5 : Product  Inputs=**  RndMeth=Zero
  Series RLC Branch1 : powerlib/Elements/Series RLC Branch  LConnTagsString=__new0  RConnTagsString=__new0  BranchType=R  Resistance=1e-6  Inductance=1e-3  SetiL0=off  InitialCurrent=0  Capacitance=1e-6  Setx0=off  InitialVoltage=0  Measurements=None
      settings: SourceProductName=Simscape Electrical
  Series RLC Branch2 : powerlib/Elements/Series RLC Branch  LConnTagsString=__new0  RConnTagsString=__new0  BranchType=R  Resistance=1e-6  Inductance=1e-3  SetiL0=off  InitialCurrent=0  Capacitance=1e-6  Setx0=off  InitialVoltage=0  Measurements=None
      settings: SourceProductName=Simscape Electrical
  Series RLC Branch6 : powerlib/Elements/Series RLC Branch  LConnTagsString=__new0  RConnTagsString=__new0  BranchType=R  Resistance=1e6  Inductance=1e-3  SetiL0=off  InitialCurrent=0  Capacitance=1e-6  Setx0=off  InitialVoltage=0  Measurements=None
      settings: SourceProductName=Simscape Electrical
  Sum1 : Sum  Inputs=++|
  Voltage Measurement1 : powerlib/Measurements/Voltage Measurement  PhasorSimulation=on  OutputType=Complex  PSBequivalent=0
      settings: SourceProductName=Simscape Electrical
  S+ : PMIOPort  Side=Left
  S- : PMIOPort  Port=2  Side=Left
  L+ : PMIOPort  Port=3  Side=Right
  L- : PMIOPort  Port=4  Side=Right
  wires:
  Sum1/1 -> Product4/3
  [I2] -> Controlled Current Source1/1
  [V1] -> Controlled Voltage Source2/1
  Constant1/1 -> Sum1/2
  Product5/1 -> Memory/1
  Product4/1 -> Memory1/1
  [Is] -> Product4/1
  Current Measurement1/1 -> [Is]
  Tap/1 -> Gain2/1
  Gain2/1 -> Sum1/1, Product4/2, Gain4/1
  Gain4/1 -> Product5/2
  [Vp] -> Product5/1
  Voltage Measurement1/1 -> [Vp]
  Memory/1 -> [V1]
  Memory1/1 -> [I2]
  connections:
  Series RLC Branch6/LConn1 -- Controlled Current Source1/RConn1 -- S-/RConn1 -- Voltage Measurement1/LConn2 -- L-/RConn1
  Controlled Voltage Source2/RConn1 -- Series RLC Branch1/LConn1
  Current Measurement1/RConn1 -- Series RLC Branch6/RConn1 -- Controlled Current Source1/LConn1 -- Series RLC Branch2/RConn1
  Controlled Voltage Source2/LConn1 -- Current Measurement1/LConn1
  Voltage Measurement1/LConn1 -- Series RLC Branch1/RConn1 -- S+/RConn1
  Series RLC Branch2/LConn1 -- L+/RConn1

== system IEEE34bus_v2019b_Phasor_DPL_ZIPload/Regulator 2/Single Phase SVR_C/Voltage Regulator Control/Tap Changer Control ==
  "Up " : Inport
  "Down " : Inport  Port=2
  Constant : Constant  Value=-1
  Constant1 : Constant
  Determine tap position : Subsystem
  Edge Detector : Subsystem  DialogController=POWERSYS.PowerSysDialog  mask(Edge Detector){model=Rising, ic=0}
      mask prompts: model "Edge:"; ic "Input at t = -eps:"
      mask help:
      | This block compares its present input to its previous input.
      |
      | If the input  is a logic signal (TRUE (1) or FALSE (0), the output is a one-step boolean signal TRUE  when  the specified edge (Rising, Falling or Either)  is detected.
      |
      | This block can also be used to detect the slope polarity of a continuous signal. For example, if the specified edge is  "Rising", the output is TRUE as long as the slope of the input signal is positive.
      |
      | The input value at time preceding t=0 is specified by the parameter "Input at t=-eps"
      mask init: same as IEEE34bus_v2019b_Phasor_DPL_ZIPload/Regulator 1/Single Phase SVR_A/Voltage Regulator Control/Tap Changer Control/Edge Detector
      mask Help: This block is part of a subset of blocks in the Extras library that does not have documentation associated with it, other than the block mask description.
      mask TypeOptions model: Rising | Falling | Either
      mask Display: plot(0,0,100,100, X1,Y1,X2,Y2,X3,Y3,X4,Y4);
  Logical Operator : Logic  Operator=OR  AllPortsSameDT=off
  Logical Operator1 : Logic  AllPortsSameDT=off
  Mechanical Delay : TransportDelay  DelayTime=MecDelay  InitialOutput=InitialPosition  BufferSize=5120
  Memory : Memory  InitialCondition=1  InheritSampleTime=on
  Relational Operator : RelationalOperator  Operator===  OutDataTypeStr=float('double')  RndMeth=Nearest
  Switch : Switch  Threshold=0.5  SaturateOnIntegerOverflow=on
  TapNo : Outport  VectorParamsAs1DForOutWhenUnconnected=off
  Ready : Outport  Port=2  VectorParamsAs1DForOutWhenUnconnected=off
  wires:
  Mechanical Delay/1 -> TapNo/1, Relational Operator/2
  Logical Operator1/1 -> Determine tap position/Trigger
  "Up "/1 -> Logical Operator/1
  "Down "/1 -> Logical Operator/2, Switch/2
  Constant/1 -> Switch/1
  Constant1/1 -> Switch/3
  Switch/1 -> Determine tap position/1(NewTap)
  Determine tap position/1(TapNo) -> Mechanical Delay/1, Relational Operator/1
  Relational Operator/1 -> Memory/1
  Memory/1 -> Logical Operator1/1, Ready/1
  Logical Operator/1 -> Edge Detector/1(In)
  Edge Detector/1(Out) -> Logical Operator1/2

== system IEEE34bus_v2019b_Phasor_DPL_ZIPload/Regulator 2/Single Phase SVR_C/Voltage Regulator Control/Voltage regulator ==
  Vmes (pu) : Inport
  Ready : Inport  Port=2
  RegOn : Inport  Port=3
  Dead Zone : DeadZone  LowerValue=-DeadBand/2  UpperValue=+DeadBand/2  SaturateOnIntegerOverflow=on
  Discrete Variable Time Delay : powerlib_meascontrol/Additional Components/Discrete Variable Time Delay  MaxDelay=3/60+Ts  InitialValue=1  Ts=Ts  DFT=on
      settings: SourceProductName=Simscape Electrical  SourceProductBaseCode=PS
  Logical Operator : Logic  AllPortsSameDT=off
  Logical Operator1 : Logic  AllPortsSameDT=off
  On Delay : powerlib_meascontrol/Logic/On Delay  DelayType=On delay  delay=TimeDelay  ic=0  Ts=Ts
      settings: SourceProductName=Simscape Electrical
  On Delay1 : powerlib_meascontrol/Logic/On Delay  DelayType=On delay  delay=TimeDelay  ic=0  Ts=Ts
      settings: SourceProductName=Simscape Electrical
  Relational Operator : RelationalOperator  Operator=>  RndMeth=Nearest
  Relational Operator1 : RelationalOperator  Operator=<  RndMeth=Nearest
  Sum : Sum  Inputs=|+-  SaturateOnIntegerOverflow=on
  Switch : Switch  Threshold=1.5  SaturateOnIntegerOverflow=on
  Vref : Constant  Value=Vref
  Vref1 : Constant  Value=0
  Vref2 : Constant  Value=0
  Vref3 : Constant  Value=0
  Vref4 : Constant  Value=3/60
  Up : Outport  VectorParamsAs1DForOutWhenUnconnected=off
  Down : Outport  Port=2  VectorParamsAs1DForOutWhenUnconnected=off
  wires:
  Vref2/1 -> Switch/3
  RegOn/1 -> Switch/2
  Switch/1 -> Dead Zone/1
  Sum/1 -> Switch/1
  Vref/1 -> Sum/1
  Vmes (pu)/1 -> Sum/2
  Dead Zone/1 -> Relational Operator1/1, Relational Operator/1
  Vref1/1 -> Relational Operator/2
  Relational Operator/1 -> Logical Operator/1
  Ready/1 -> Discrete Variable Time Delay/1
  Logical Operator/1 -> On Delay/1
  On Delay/1 -> Up/1
  Relational Operator1/1 -> Logical Operator1/2
  Logical Operator1/1 -> On Delay1/1
  On Delay1/1 -> Down/1
  Vref3/1 -> Relational Operator1/2
  Discrete Variable Time Delay/1 -> Logical Operator1/1, Logical Operator/2
  Vref4/1 -> Discrete Variable Time Delay/2

== system IEEE34bus_v2019b_Phasor_DPL_ZIPload/Regulator 1/Single Phase SVR_A/Voltage Regulator Control/Tap Changer Control/Determine tap position ==
  NewTap : Inport
  Trigger : TriggerPort  VariantControl=Variant
  Memory : Memory  InitialCondition=InitialPosition  InheritSampleTime=on
  Saturation : Saturate  UpperLimit=MinMaxTap(2)  LowerLimit=MinMaxTap(1)
  Sum : Sum  Inputs=|++  SaturateOnIntegerOverflow=on
  TapNo : Outport  InitialOutput=InitialPosition  VectorParamsAs1DForOutWhenUnconnected=off
  wires:
  NewTap/1 -> Sum/1
  Sum/1 -> Saturation/1
  Memory/1 -> Sum/2
  Saturation/1 -> TapNo/1, Memory/1

== system IEEE34bus_v2019b_Phasor_DPL_ZIPload/Regulator 1/Single Phase SVR_A/Voltage Regulator Control/Tap Changer Control/Edge Detector ==
  note: Edge or Slope Detector
  In : Inport
  Constant1 : Constant  Value=model
  Demux : Demux  Outputs=2
  Logical Operator1 : Logic  Operator=OR
  Memory : Memory  InitialCondition=ic  LinearizeAsDelay=on
  Multiport Switch : MultiPortSwitch  SaturateOnIntegerOverflow=on
  NEGATIVE Edge : Subsystem  TreatAsAtomicUnit=on
  POSITIVE Edge : Subsystem  TreatAsAtomicUnit=on
  either edge : Constant  Value=[1 1]
  neg. edge : Constant  Value=[0 1]
  pos. edge : Constant  Value=[1 0]
  Out : Outport  VectorParamsAs1DForOutWhenUnconnected=off
  wires:
  either edge/1 -> Multiport Switch/4
  Demux/2 -> NEGATIVE Edge/Enable
  Demux/1 -> POSITIVE Edge/Enable
  Multiport Switch/1 -> Demux/1
  Constant1/1 -> Multiport Switch/1
  neg. edge/1 -> Multiport Switch/3
  pos. edge/1 -> Multiport Switch/2
  In/1 -> Memory/1, NEGATIVE Edge/1(IN), POSITIVE Edge/1(IN)
  Memory/1 -> NEGATIVE Edge/2(IN previous), POSITIVE Edge/2(IN previous)
  POSITIVE Edge/1(OUT) -> Logical Operator1/1
  NEGATIVE Edge/1(OUT) -> Logical Operator1/2
  Logical Operator1/1 -> Out/1

== system IEEE34bus_v2019b_Phasor_DPL_ZIPload/Regulator 1/Single Phase SVR_B/Voltage Regulator Control/Tap Changer Control/Determine tap position ==
  NewTap : Inport
  Trigger : TriggerPort  VariantControl=Variant
  Memory : Memory  InitialCondition=InitialPosition  InheritSampleTime=on
  Saturation : Saturate  UpperLimit=MinMaxTap(2)  LowerLimit=MinMaxTap(1)
  Sum : Sum  Inputs=|++  SaturateOnIntegerOverflow=on
  TapNo : Outport  InitialOutput=InitialPosition  VectorParamsAs1DForOutWhenUnconnected=off
  wires:
  NewTap/1 -> Sum/1
  Sum/1 -> Saturation/1
  Memory/1 -> Sum/2
  Saturation/1 -> TapNo/1, Memory/1

== system IEEE34bus_v2019b_Phasor_DPL_ZIPload/Regulator 1/Single Phase SVR_B/Voltage Regulator Control/Tap Changer Control/Edge Detector ==
  note: Edge or Slope Detector
  In : Inport
  Constant1 : Constant  Value=model
  Demux : Demux  Outputs=2
  Logical Operator1 : Logic  Operator=OR
  Memory : Memory  InitialCondition=ic  LinearizeAsDelay=on
  Multiport Switch : MultiPortSwitch  SaturateOnIntegerOverflow=on
  NEGATIVE Edge : Subsystem  TreatAsAtomicUnit=on
  POSITIVE Edge : Subsystem  TreatAsAtomicUnit=on
  either edge : Constant  Value=[1 1]
  neg. edge : Constant  Value=[0 1]
  pos. edge : Constant  Value=[1 0]
  Out : Outport  VectorParamsAs1DForOutWhenUnconnected=off
  wires:
  either edge/1 -> Multiport Switch/4
  Demux/2 -> NEGATIVE Edge/Enable
  Demux/1 -> POSITIVE Edge/Enable
  Multiport Switch/1 -> Demux/1
  Constant1/1 -> Multiport Switch/1
  neg. edge/1 -> Multiport Switch/3
  pos. edge/1 -> Multiport Switch/2
  In/1 -> Memory/1, NEGATIVE Edge/1(IN), POSITIVE Edge/1(IN)
  Memory/1 -> NEGATIVE Edge/2(IN previous), POSITIVE Edge/2(IN previous)
  POSITIVE Edge/1(OUT) -> Logical Operator1/1
  NEGATIVE Edge/1(OUT) -> Logical Operator1/2
  Logical Operator1/1 -> Out/1

== system IEEE34bus_v2019b_Phasor_DPL_ZIPload/Regulator 1/Single Phase SVR_C/Voltage Regulator Control/Tap Changer Control/Determine tap position ==
  NewTap : Inport
  Trigger : TriggerPort  VariantControl=Variant
  Memory : Memory  InitialCondition=InitialPosition  InheritSampleTime=on
  Saturation : Saturate  UpperLimit=MinMaxTap(2)  LowerLimit=MinMaxTap(1)
  Sum : Sum  Inputs=|++  SaturateOnIntegerOverflow=on
  TapNo : Outport  InitialOutput=InitialPosition  VectorParamsAs1DForOutWhenUnconnected=off
  wires:
  NewTap/1 -> Sum/1
  Sum/1 -> Saturation/1
  Memory/1 -> Sum/2
  Saturation/1 -> TapNo/1, Memory/1

== system IEEE34bus_v2019b_Phasor_DPL_ZIPload/Regulator 1/Single Phase SVR_C/Voltage Regulator Control/Tap Changer Control/Edge Detector ==
  note: Edge or Slope Detector
  In : Inport
  Constant1 : Constant  Value=model
  Demux : Demux  Outputs=2
  Logical Operator1 : Logic  Operator=OR
  Memory : Memory  InitialCondition=ic  LinearizeAsDelay=on
  Multiport Switch : MultiPortSwitch  SaturateOnIntegerOverflow=on
  NEGATIVE Edge : Subsystem  TreatAsAtomicUnit=on
  POSITIVE Edge : Subsystem  TreatAsAtomicUnit=on
  either edge : Constant  Value=[1 1]
  neg. edge : Constant  Value=[0 1]
  pos. edge : Constant  Value=[1 0]
  Out : Outport  VectorParamsAs1DForOutWhenUnconnected=off
  wires:
  either edge/1 -> Multiport Switch/4
  Demux/2 -> NEGATIVE Edge/Enable
  Demux/1 -> POSITIVE Edge/Enable
  Multiport Switch/1 -> Demux/1
  Constant1/1 -> Multiport Switch/1
  neg. edge/1 -> Multiport Switch/3
  pos. edge/1 -> Multiport Switch/2
  In/1 -> Memory/1, NEGATIVE Edge/1(IN), POSITIVE Edge/1(IN)
  Memory/1 -> NEGATIVE Edge/2(IN previous), POSITIVE Edge/2(IN previous)
  POSITIVE Edge/1(OUT) -> Logical Operator1/1
  NEGATIVE Edge/1(OUT) -> Logical Operator1/2
  Logical Operator1/1 -> Out/1

== system IEEE34bus_v2019b_Phasor_DPL_ZIPload/Regulator 2/Single Phase SVR_A/Voltage Regulator Control/Tap Changer Control/Determine tap position ==
  NewTap : Inport
  Trigger : TriggerPort  VariantControl=Variant
  Memory : Memory  InitialCondition=InitialPosition  InheritSampleTime=on
  Saturation : Saturate  UpperLimit=MinMaxTap(2)  LowerLimit=MinMaxTap(1)
  Sum : Sum  Inputs=|++  SaturateOnIntegerOverflow=on
  TapNo : Outport  InitialOutput=InitialPosition  VectorParamsAs1DForOutWhenUnconnected=off
  wires:
  NewTap/1 -> Sum/1
  Sum/1 -> Saturation/1
  Memory/1 -> Sum/2
  Saturation/1 -> TapNo/1, Memory/1

== system IEEE34bus_v2019b_Phasor_DPL_ZIPload/Regulator 2/Single Phase SVR_A/Voltage Regulator Control/Tap Changer Control/Edge Detector ==
  note: Edge or Slope Detector
  In : Inport
  Constant1 : Constant  Value=model
  Demux : Demux  Outputs=2
  Logical Operator1 : Logic  Operator=OR
  Memory : Memory  InitialCondition=ic  LinearizeAsDelay=on
  Multiport Switch : MultiPortSwitch  SaturateOnIntegerOverflow=on
  NEGATIVE Edge : Subsystem  TreatAsAtomicUnit=on
  POSITIVE Edge : Subsystem  TreatAsAtomicUnit=on
  either edge : Constant  Value=[1 1]
  neg. edge : Constant  Value=[0 1]
  pos. edge : Constant  Value=[1 0]
  Out : Outport  VectorParamsAs1DForOutWhenUnconnected=off
  wires:
  either edge/1 -> Multiport Switch/4
  Demux/2 -> NEGATIVE Edge/Enable
  Demux/1 -> POSITIVE Edge/Enable
  Multiport Switch/1 -> Demux/1
  Constant1/1 -> Multiport Switch/1
  neg. edge/1 -> Multiport Switch/3
  pos. edge/1 -> Multiport Switch/2
  In/1 -> Memory/1, NEGATIVE Edge/1(IN), POSITIVE Edge/1(IN)
  Memory/1 -> NEGATIVE Edge/2(IN previous), POSITIVE Edge/2(IN previous)
  POSITIVE Edge/1(OUT) -> Logical Operator1/1
  NEGATIVE Edge/1(OUT) -> Logical Operator1/2
  Logical Operator1/1 -> Out/1

== system IEEE34bus_v2019b_Phasor_DPL_ZIPload/Regulator 2/Single Phase SVR_B/Voltage Regulator Control/Tap Changer Control/Determine tap position ==
  NewTap : Inport
  Trigger : TriggerPort  VariantControl=Variant
  Memory : Memory  InitialCondition=InitialPosition  InheritSampleTime=on
  Saturation : Saturate  UpperLimit=MinMaxTap(2)  LowerLimit=MinMaxTap(1)
  Sum : Sum  Inputs=|++  SaturateOnIntegerOverflow=on
  TapNo : Outport  InitialOutput=InitialPosition  VectorParamsAs1DForOutWhenUnconnected=off
  wires:
  NewTap/1 -> Sum/1
  Sum/1 -> Saturation/1
  Memory/1 -> Sum/2
  Saturation/1 -> TapNo/1, Memory/1

== system IEEE34bus_v2019b_Phasor_DPL_ZIPload/Regulator 2/Single Phase SVR_B/Voltage Regulator Control/Tap Changer Control/Edge Detector ==
  note: Edge or Slope Detector
  In : Inport
  Constant1 : Constant  Value=model
  Demux : Demux  Outputs=2
  Logical Operator1 : Logic  Operator=OR
  Memory : Memory  InitialCondition=ic  LinearizeAsDelay=on
  Multiport Switch : MultiPortSwitch  SaturateOnIntegerOverflow=on
  NEGATIVE Edge : Subsystem  TreatAsAtomicUnit=on
  POSITIVE Edge : Subsystem  TreatAsAtomicUnit=on
  either edge : Constant  Value=[1 1]
  neg. edge : Constant  Value=[0 1]
  pos. edge : Constant  Value=[1 0]
  Out : Outport  VectorParamsAs1DForOutWhenUnconnected=off
  wires:
  either edge/1 -> Multiport Switch/4
  Demux/2 -> NEGATIVE Edge/Enable
  Demux/1 -> POSITIVE Edge/Enable
  Multiport Switch/1 -> Demux/1
  Constant1/1 -> Multiport Switch/1
  neg. edge/1 -> Multiport Switch/3
  pos. edge/1 -> Multiport Switch/2
  In/1 -> Memory/1, NEGATIVE Edge/1(IN), POSITIVE Edge/1(IN)
  Memory/1 -> NEGATIVE Edge/2(IN previous), POSITIVE Edge/2(IN previous)
  POSITIVE Edge/1(OUT) -> Logical Operator1/1
  NEGATIVE Edge/1(OUT) -> Logical Operator1/2
  Logical Operator1/1 -> Out/1

== system IEEE34bus_v2019b_Phasor_DPL_ZIPload/Regulator 2/Single Phase SVR_C/Voltage Regulator Control/Tap Changer Control/Determine tap position ==
  NewTap : Inport
  Trigger : TriggerPort  VariantControl=Variant
  Memory : Memory  InitialCondition=InitialPosition  InheritSampleTime=on
  Saturation : Saturate  UpperLimit=MinMaxTap(2)  LowerLimit=MinMaxTap(1)
  Sum : Sum  Inputs=|++  SaturateOnIntegerOverflow=on
  TapNo : Outport  InitialOutput=InitialPosition  VectorParamsAs1DForOutWhenUnconnected=off
  wires:
  NewTap/1 -> Sum/1
  Sum/1 -> Saturation/1
  Memory/1 -> Sum/2
  Saturation/1 -> TapNo/1, Memory/1

== system IEEE34bus_v2019b_Phasor_DPL_ZIPload/Regulator 2/Single Phase SVR_C/Voltage Regulator Control/Tap Changer Control/Edge Detector ==
  note: Edge or Slope Detector
  In : Inport
  Constant1 : Constant  Value=model
  Demux : Demux  Outputs=2
  Logical Operator1 : Logic  Operator=OR
  Memory : Memory  InitialCondition=ic  LinearizeAsDelay=on
  Multiport Switch : MultiPortSwitch  SaturateOnIntegerOverflow=on
  NEGATIVE Edge : Subsystem  TreatAsAtomicUnit=on
  POSITIVE Edge : Subsystem  TreatAsAtomicUnit=on
  either edge : Constant  Value=[1 1]
  neg. edge : Constant  Value=[0 1]
  pos. edge : Constant  Value=[1 0]
  Out : Outport  VectorParamsAs1DForOutWhenUnconnected=off
  wires:
  either edge/1 -> Multiport Switch/4
  Demux/2 -> NEGATIVE Edge/Enable
  Demux/1 -> POSITIVE Edge/Enable
  Multiport Switch/1 -> Demux/1
  Constant1/1 -> Multiport Switch/1
  neg. edge/1 -> Multiport Switch/3
  pos. edge/1 -> Multiport Switch/2
  In/1 -> Memory/1, NEGATIVE Edge/1(IN), POSITIVE Edge/1(IN)
  Memory/1 -> NEGATIVE Edge/2(IN previous), POSITIVE Edge/2(IN previous)
  POSITIVE Edge/1(OUT) -> Logical Operator1/1
  NEGATIVE Edge/1(OUT) -> Logical Operator1/2
  Logical Operator1/1 -> Out/1

== system IEEE34bus_v2019b_Phasor_DPL_ZIPload/Regulator 1/Single Phase SVR_A/Voltage Regulator Control/Tap Changer Control/Edge Detector/NEGATIVE Edge ==
  IN : Inport
  IN previous : Inport  Port=2
  Enable : EnablePort  PropagateVarSize=During execution
  Relational Operator1 : RelationalOperator  Operator=>  RndMeth=Nearest  InputSameDT=on
  OUT : Outport  VectorParamsAs1DForOutWhenUnconnected=off
  wires:
  IN/1 -> Relational Operator1/2
  IN previous/1 -> Relational Operator1/1
  Relational Operator1/1 -> OUT/1

== system IEEE34bus_v2019b_Phasor_DPL_ZIPload/Regulator 1/Single Phase SVR_A/Voltage Regulator Control/Tap Changer Control/Edge Detector/POSITIVE Edge ==
  IN : Inport
  IN previous : Inport  Port=2
  Enable : EnablePort  PropagateVarSize=During execution
  Relational Operator1 : RelationalOperator  Operator=>  RndMeth=Nearest  InputSameDT=on
  OUT : Outport  VectorParamsAs1DForOutWhenUnconnected=off
  wires:
  IN/1 -> Relational Operator1/1
  IN previous/1 -> Relational Operator1/2
  Relational Operator1/1 -> OUT/1

== system IEEE34bus_v2019b_Phasor_DPL_ZIPload/Regulator 1/Single Phase SVR_B/Voltage Regulator Control/Tap Changer Control/Edge Detector/NEGATIVE Edge ==
  IN : Inport
  IN previous : Inport  Port=2
  Enable : EnablePort  PropagateVarSize=During execution
  Relational Operator1 : RelationalOperator  Operator=>  RndMeth=Nearest  InputSameDT=on
  OUT : Outport  VectorParamsAs1DForOutWhenUnconnected=off
  wires:
  IN/1 -> Relational Operator1/2
  IN previous/1 -> Relational Operator1/1
  Relational Operator1/1 -> OUT/1

== system IEEE34bus_v2019b_Phasor_DPL_ZIPload/Regulator 1/Single Phase SVR_B/Voltage Regulator Control/Tap Changer Control/Edge Detector/POSITIVE Edge ==
  IN : Inport
  IN previous : Inport  Port=2
  Enable : EnablePort  PropagateVarSize=During execution
  Relational Operator1 : RelationalOperator  Operator=>  RndMeth=Nearest  InputSameDT=on
  OUT : Outport  VectorParamsAs1DForOutWhenUnconnected=off
  wires:
  IN/1 -> Relational Operator1/1
  IN previous/1 -> Relational Operator1/2
  Relational Operator1/1 -> OUT/1

== system IEEE34bus_v2019b_Phasor_DPL_ZIPload/Regulator 1/Single Phase SVR_C/Voltage Regulator Control/Tap Changer Control/Edge Detector/NEGATIVE Edge ==
  IN : Inport
  IN previous : Inport  Port=2
  Enable : EnablePort  PropagateVarSize=During execution
  Relational Operator1 : RelationalOperator  Operator=>  RndMeth=Nearest  InputSameDT=on
  OUT : Outport  VectorParamsAs1DForOutWhenUnconnected=off
  wires:
  IN/1 -> Relational Operator1/2
  IN previous/1 -> Relational Operator1/1
  Relational Operator1/1 -> OUT/1
